simulink model "districtScreeningSimEvents"  (R2026a)
settings: Solver=VariableStepAuto  StopTime=576000
PreLoadFcn:
  | buildEntityBus();
values from neighbouring files (symbols this model uses):
  n = workers    [monteCarloQueueing.m]    (also in referenceQueueingModel.m = 1; sweepDistrictScenarios.m)
undefined symbols (not defined in the file or in its folder): m
settings Model: Creator=91740  LastModifiedBy=91740

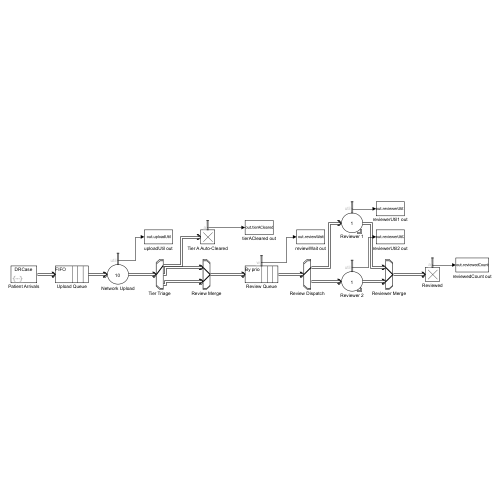
[thumbnail: Simulink's stored preview of the top-level diagram]
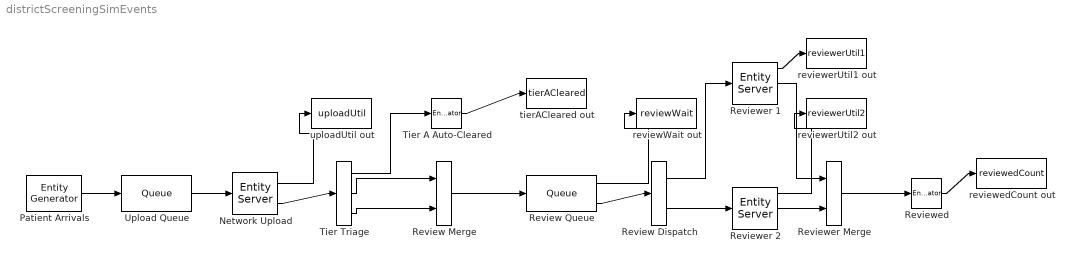
== system districtScreeningSimEvents ==
  Network Upload : EntityServer  InputPortMessageModes=m  OutputPortMessageModes=n,m  Capacity=10  ServiceTimeSource=MATLAB action  ServiceTimeAction=dt = -29.6*log(rand());  Utilization=on
      settings: OutputPortMap=o5,o9
  Patient Arrivals : EntityGenerator  OutputPortMessageModes=m  TimeSource=MATLAB action  IntergenerationTimeAction=dt = -72*log(rand());  GenerateAction=|  EntityType=Bus object  EntityTypeName=DRCase
      | u = rand();
      | if u < 0.700000
      |   entity.prio = 1;
      | elseif u < 0.900000
      |   entity.prio = 2;
      | else
      |   entity.prio = 3;
      | end
  Review Dispatch : EntityOutputSwitch  InputPortMessageModes=m  OutputPortMessageModes=m,m  SwitchAttributeName=Attribute1
  Review Merge : EntityInputSwitch  InputPortMessageModes=m,m  OutputPortMessageModes=m
  Review Queue : Queue  InputPortMessageModes=m  OutputPortMessageModes=n,m  Capacity=inf  QueueType=Priority  PrioritySource=prio  SortingDirection=Descending  AverageWait=on
      settings: OutputPortMap=o2,o5
  Reviewed : EntityTerminator  InputPortMessageModes=m  NumberEntitiesArrived=on
      settings: OutputPortMap=o0
  Reviewer 1 : EntityServer  InputPortMessageModes=m  OutputPortMessageModes=n,m,m  Capacity=1  ServiceTimeSource=MATLAB action  ServiceTimeAction=|  PermitPreemptionBasedOnAttribute=on  SortingAttributeName=prio  SortingDirection=Descending  WriteResidualTimeToAttribute=on  ResidualTimeAttributeName=residual  Utilization=on
      | if entity.prio == 3
      |   dt = -240*log(rand());
      | else
      |   dt = -30*log(rand());
      | end
      settings: OutputPortMap=o5,o9,o10
  Reviewer 2 : EntityServer  InputPortMessageModes=m  OutputPortMessageModes=n,m,m  Capacity=1  ServiceTimeSource=MATLAB action  ServiceTimeAction=|  PermitPreemptionBasedOnAttribute=on  SortingAttributeName=prio  SortingDirection=Descending  WriteResidualTimeToAttribute=on  ResidualTimeAttributeName=residual  Utilization=on
      | if entity.prio == 3
      |   dt = -240*log(rand());
      | else
      |   dt = -30*log(rand());
      | end
      settings: OutputPortMap=o5,o9,o10
  Reviewer Merge : EntityInputSwitch  InputPortMessageModes=m,m  OutputPortMessageModes=m
  Tier A Auto-Cleared : EntityTerminator  InputPortMessageModes=m  NumberEntitiesArrived=on
      settings: OutputPortMap=o0
  Tier Triage : EntityOutputSwitch  InputPortMessageModes=m  OutputPortMessageModes=m,m,m  NumberOutputPorts=3  SwitchingCriterion=From attribute  SwitchAttributeName=prio
      settings: OutputPortMap=o0,o1,o2
  Upload Queue : Queue  InputPortMessageModes=m  OutputPortMessageModes=m  Capacity=inf
  reviewWait out : ToWorkspace  VariableName=reviewWait  SaveFormat=Timeseries  SampleTime=-1
  reviewedCount out : ToWorkspace  VariableName=reviewedCount  SaveFormat=Timeseries  SampleTime=-1
  reviewerUtil1 out : ToWorkspace  VariableName=reviewerUtil1  SaveFormat=Timeseries  SampleTime=-1
  reviewerUtil2 out : ToWorkspace  VariableName=reviewerUtil2  SaveFormat=Timeseries  SampleTime=-1
  tierACleared out : ToWorkspace  VariableName=tierACleared  SaveFormat=Timeseries  SampleTime=-1
  uploadUtil out : ToWorkspace  VariableName=uploadUtil  SaveFormat=Timeseries  SampleTime=-1
  wires:
  Network Upload/1 -> uploadUtil out/1
  Tier A Auto-Cleared/1 -> tierACleared out/1
  Tier Triage/3 -> Review Merge/2
  Review Merge/1 -> Review Queue/1
  Upload Queue/1 -> Network Upload/1
  Tier Triage/2 -> Review Merge/1
  Tier Triage/1 -> Tier A Auto-Cleared/1
  Review Queue/2 -> Review Dispatch/1
  Network Upload/2 -> Tier Triage/1
  Patient Arrivals/1 -> Upload Queue/1
  Reviewer 1/1 -> reviewerUtil1 out/1
  Review Queue/1 -> reviewWait out/1
  Review Dispatch/1 -> Reviewer 1/1
  Reviewer 2/2 -> Reviewer Merge/2
  Review Dispatch/2 -> Reviewer 2/1
  Reviewer 1/2 -> Reviewer Merge/1
  Reviewed/1 -> reviewedCount out/1
  Reviewer 2/1 -> reviewerUtil2 out/1
  Reviewer Merge/1 -> Reviewed/1
